simulink model "model_sim"  (R2017b)
settings: Solver=VariableStepAuto  StartTime=0.0  StopTime=10.0  RelTol=1e-3
values from neighbouring files (symbols this model uses):
  A = zeros(5,5)    [kalmanfilter.m]    (also in model_2017.m = [[0  0   0   0                0             0   1           ; model_rough.m; model_v2.m = [[0  0   0   0             0             0   1           0  ; model_v3.m = [[0  0   0   0                0             0   1           )
  B = zeros(5,6)    [kalmanfilter.m]    (also in model_2017.m = [[0      0      0      0     ];                        [0   ; model_rough.m; model_v2.m = [[0      0      0      0     ];                        [0   ; model_v3.m = [[0      0      0      0      0      0             ];       )
  C = eye(5)    [kalmanfilter.m]    (also in model_2017.m = [[0  0   0   0   0   0   1   0   0   0   0   0]; model_rough.m; model_v2.m = [[0  0   0   0   0   0   1   0   0   0   0   0]; model_v3.m = [[0  0   0   0   0   0   1   0   0   0   0   0])
  K = []    [kalmanfilter.m]    (also in model_rough.m = place(A, B, polevec))
settings Model: Creator=Simon's  LastModifiedBy=viral
settings CodeAppCC: StateflowObjectComments=on

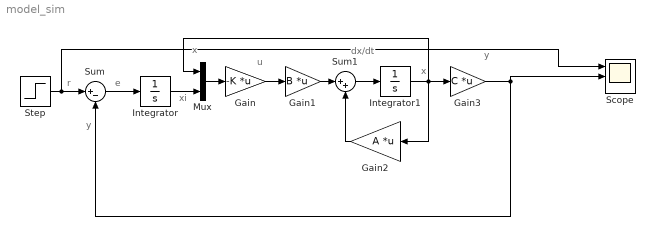
== system model_sim ==
  note: x
  note: y
  note: e
  note: xi
  note: u
  note: r
  note: y
  note: dx/dt
  note: x
  Gain : Gain  Gain=-K  Multiplication=Matrix(K*u)
  Gain1 : Gain  Gain=B  Multiplication=Matrix(K*u)
  Gain2 : Gain  Gain=A  Multiplication=Matrix(K*u)
  Gain3 : Gain  Gain=C  Multiplication=Matrix(K*u)
  Integrator : Integrator
  Integrator1 : Integrator
  Mux : Mux  Inputs=2
  Scope : Scope  NumInputPorts=3
  Step : Step  Before="[0  0 0 0 0 0]"  After=[1 0 0 0 0 0]  SampleTime=0
  Sum : Sum  Inputs=|+-
  Sum1 : Sum  Inputs=|++
  wires:
  Step/1 -> Scope/1, Sum/1
  Sum/1 -> Integrator/1
  Gain1/1 -> Sum1/1
  Sum1/1 -> Integrator1/1
  Gain2/1 -> Sum1/2
  Gain3/1 -> Sum/2, Scope/2
  Mux/1 -> Gain/1
  Integrator/1 -> Mux/2
  Integrator1/1 -> Gain2/1, Mux/1, Gain3/1
  Gain/1 -> Gain1/1
  ? -> Scope/3
